simulink model "SB4_bus_todo"  (R2024b)
settings: Solver=FixedStepDiscrete  StartTime=0.0  StopTime=1  FixedStep=0.05  RelTol=1e-3
settings Model: Creator=admin  LastModifiedBy=admin

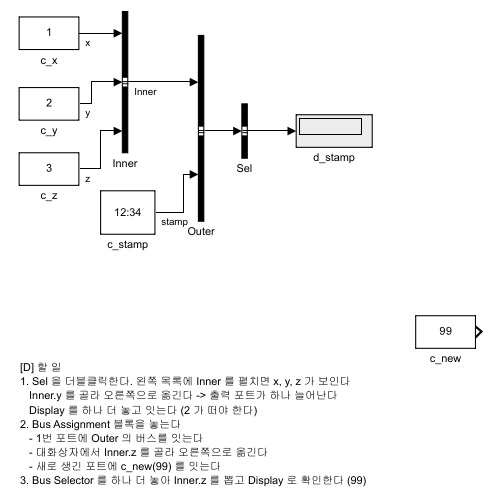
[thumbnail: Simulink's stored preview of the top-level diagram]
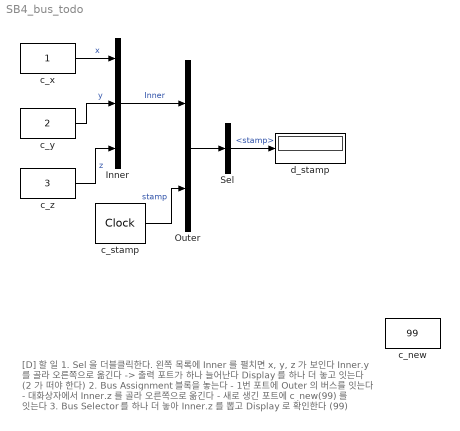
== system SB4_bus_todo ==
  note: [D] 할 일
      | 1. Sel 을 더블클릭한다. 왼쪽 목록에 Inner 를 펼치면 x, y, z 가 보인다
      |    Inner.y 를 골라 오른쪽으로 옮긴다 -> 출력 포트가 하나 늘어난다
      |    Display 를 하나 더 놓고 잇는다 (2 가 떠야 한다)
      | 2. Bus Assignment 블록을 놓는다
      |    - 1번 포트에 Outer 의 버스를 잇는다
      |    - 대화상자에서 Inner.z 를 골라 오른쪽으로 옮긴다
      |    - 새로 생긴 포트에 c_new(99) 를 잇는다
      | 3. Bus Selector 를 하나 더 놓아 Inner.z 를 뽑고 Display 로 확인한다 (99)
  Inner : BusCreator  Inputs=3
  Outer : BusCreator  Inputs=2
  Sel : BusSelector  OutputSignals=stamp
  c_new : Constant  Value=99
  c_stamp : DigitalClock  SampleTime=0.05
  c_x : Constant
  c_y : Constant  Value=2
  c_z : Constant  Value=3
  d_stamp : Display
  wires:
  c_x/1 -> Inner/1  "x"
  c_y/1 -> Inner/2  "y"
  c_stamp/1 -> Outer/2  "stamp"
  Inner/1 -> Outer/1  "Inner"
  c_z/1 -> Inner/3  "z"
  Sel/1 -> d_stamp/1  "<stamp>"
  Outer/1 -> Sel/1
